simulink model "Full_Bridge_Series_LLC_Resonant_Converters"  (R2024b)
settings: Solver=VariableStepAuto  StartTime=0.0  StopTime=10.0  RelTol=1e-3
libraries: spsDiodeLib x4, spsMosfetLib x4, spsVoltageMeasurementLib x4, spsCurrentMeasurementLib x3, spsSeriesRLCBranchLib x3, eePwmGenerator x2, spsDCVoltageSourceLib x1, spsMultiWindingTransformerLib x1, spspowerguiLib x1
settings Model: Creator=User  LastModifiedBy=User

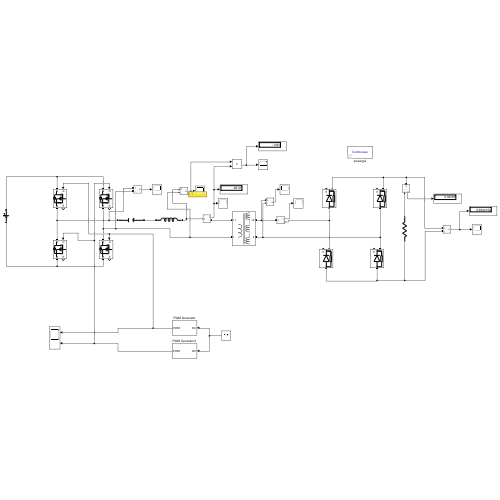
[thumbnail: Simulink's stored preview of the top-level diagram]
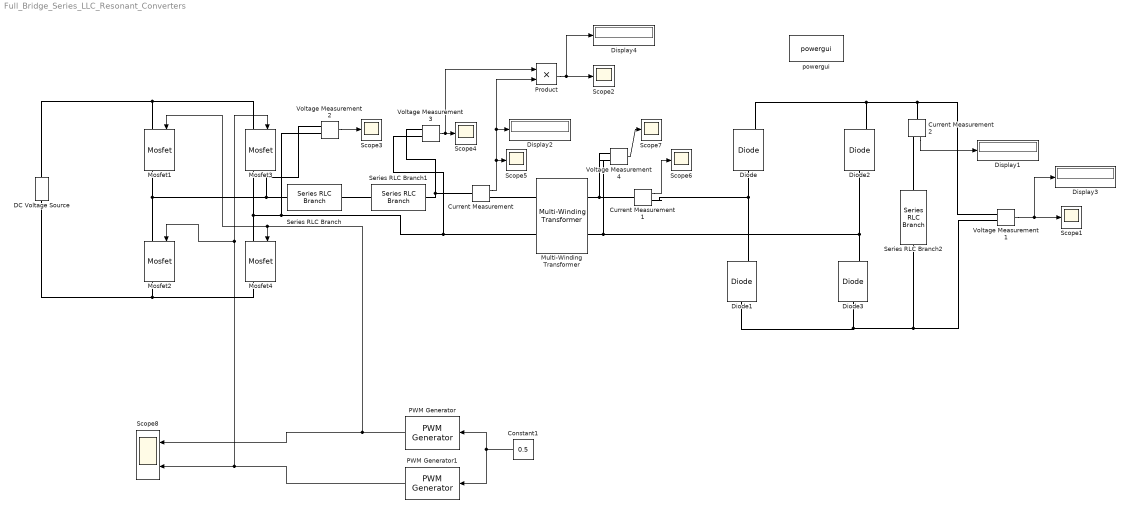
== system Full_Bridge_Series_LLC_Resonant_Converters ==
  Constant1 : Constant  Value=0.5
  Current Measurement : spsCurrentMeasurementLib/Current Measurement  PhasorSimulation=off  OutputType=Complex  PSBequivalent=0
  Current Measurement1 : spsCurrentMeasurementLib/Current Measurement  PhasorSimulation=off  OutputType=Complex  PSBequivalent=0
  Current Measurement2 : spsCurrentMeasurementLib/Current Measurement  PhasorSimulation=off  OutputType=Complex  PSBequivalent=0
  DC Voltage Source : spsDCVoltageSourceLib/DC Voltage Source  Amplitude=200  Measurements=Voltage
  Diode{,1..3} (4 alike) : spsDiodeLib/Diode  Ron=0.001  Lon=0  Vf=0  IC=0  UseSnubber=0  Rs=500  Cs=100e-12  Measurements=on
  Display{1..4} (4 alike) : Display
  Mosfet{1..4} (4 alike) : spsMosfetLib/Mosfet  Ron=0.1  Lon=0  Rd=0.01  Vfd=0  IC=0  Rs=1e5  Cs=inf  Measurements=on
  Multi-Winding Transformer : spsMultiWindingTransformerLib/Multi-Winding Transformer  LeftWindings=1  RightWindings=1  TappedWindings=no taps  NumberOfTaps=2  SetSaturation=off  Hysteresis=off  DataFile='hysteresis.mat'  Measurements=None  UNITS=SI  NominalPower=[300 50e3]  NominalVoltages=[200 20000]  WindingResistances=[0 0]  WindingInductances=[0 0]  Rm=1.3824e7  Lm=18.09  Saturation=[0 0;0.25 0.1459;104.17 0.18481]  SpecifyInitialFlux=off  InitialFlux=0  BreakLoop=off  DiscreteSolver=Trapezoidal iterative  DataType=on  TransfoNumber=1
  PWM Generator : eePwmGenerator/PWM Generator  CarrCount=Up  Tper=2e-5  Tdelay=0  Ts=0
  PWM Generator1 : eePwmGenerator/PWM Generator  CarrCount=Up  Tper=2e-5  Tdelay=1e-5  Ts=0
  Product : Product
  Scope{1..7} (7 alike) : Scope
  Scope8 : Scope  NumInputPorts=2
  Series RLC Branch : spsSeriesRLCBranchLib/Series RLC Branch  LConnTagsString=__new0  RConnTagsString=__new0  BranchType=C  Resistance=1  Inductance=33e-3  SetiL0=off  InitialCurrent=0  Capacitance=49.09e-9  Setx0=off  InitialVoltage=0  Measurements=None
  Series RLC Branch1 : spsSeriesRLCBranchLib/Series RLC Branch  LConnTagsString=__new0  RConnTagsString=__new0  BranchType=L  Resistance=1  Inductance=206.4e-6  SetiL0=off  InitialCurrent=0  Capacitance=49.09e-9  Setx0=off  InitialVoltage=0  Measurements=None
  Series RLC Branch2 : spsSeriesRLCBranchLib/Series RLC Branch  LConnTagsString=__new0  RConnTagsString=__new0  BranchType=R  Resistance=750e3  Inductance=206.4e-6  SetiL0=off  InitialCurrent=0  Capacitance=49.09e-9  Setx0=off  InitialVoltage=0  Measurements=None
  Voltage Measurement{1..4} (4 alike) : spsVoltageMeasurementLib/Voltage Measurement  PhasorSimulation=off  OutputType=Complex  PSBequivalent=0
  powergui : spspowerguiLib/powergui  Priority=1  SimulationMode=Continuous  SampleTime=50e-6  frequency=60  Iterations=50  frequencyindice=0  Pbase=100e6  ErrMax=1e-4  UnitsV=kV  UnitsW=MW  buscounter=0  FunctionMessages=off  echomessages=off  EnableUseOfTLC=off  CurrentSourceSwitches=off  DisableSnubberDevices=off  DisableRonSwitches=off  DisableVfSwitches=off  DisplayEquations=off  AutomaticDiscreteSolvers=off  SolverType=Tustin/Backward Euler (TBE)  Interpol=off  ExternalGateDelay=off  methode=off  Ts=100  x0status=blocks  SPID=on  SwTol=0  HookPort=off  NonlinearTolerance=0  nMaxIteration=15  ContinueOnMaxIteration=off  RestoreLinks=warning  ResistiveCurrentMeasurement=off  Frange=[0:2:500]  Ylog=off  Xlog=on  ShowGrid=off  save=off  variable=ZData  structure=0  ZoomFFT=off  StartTime=0.0  cycles=1  DisplayStyle=1  fundamental=60  FreqAxis=off  MaxFrequency=1000  frequencyindicesteady=1  RmsSteady=1  display=off
  wires:
  PWM Generator1/1 -> Mosfet2/1, Mosfet3/1, Scope8/2
  Voltage Measurement1/1 -> Display3/1, Scope1/1
  Voltage Measurement3/1 -> Product/1, Scope4/1
  Voltage Measurement2/1 -> Scope3/1
  Current Measurement/1 -> Product/2, Display2/1, Scope5/1
  Current Measurement1/1 -> Scope6/1
  Voltage Measurement4/1 -> Scope7/1
  Current Measurement2/1 -> Display1/1
  PWM Generator/1 -> Mosfet4/1, Mosfet1/1, Scope8/1
  Constant1/1 -> PWM Generator1/1, PWM Generator/1
  Product/1 -> Display4/1, Scope2/1
  connections:
  Mosfet3/LConn1 -- Mosfet1/LConn1 -- DC Voltage Source/RConn1
  Mosfet1/RConn1 -- Voltage Measurement2/LConn1 -- Series RLC Branch/LConn1 -- Mosfet2/LConn1
  Mosfet3/RConn1 -- Voltage Measurement3/LConn2 -- Multi-Winding Transformer/LConn2 -- Voltage Measurement2/LConn2 -- Mosfet4/LConn1
  Mosfet4/RConn1 -- DC Voltage Source/LConn1 -- Mosfet2/RConn1
  Diode1/RConn1 -- Current Measurement1/RConn1 -- Diode/LConn1
  Diode3/RConn1 -- Multi-Winding Transformer/RConn2 -- Voltage Measurement4/LConn2 -- Diode2/LConn1
  Diode1/LConn1 -- Series RLC Branch2/RConn1 -- Voltage Measurement1/LConn2 -- Diode3/LConn1
  Diode2/RConn1 -- Current Measurement2/LConn1 -- Voltage Measurement1/LConn1 -- Diode/RConn1
  Series RLC Branch1/RConn1 -- Current Measurement/LConn1 -- Voltage Measurement3/LConn1
  Series RLC Branch1/LConn1 -- Series RLC Branch/RConn1
  Current Measurement/RConn1 -- Multi-Winding Transformer/LConn1
  Current Measurement1/LConn1 -- Voltage Measurement4/LConn1 -- Multi-Winding Transformer/RConn1
  Current Measurement2/RConn1 -- Series RLC Branch2/LConn1
